simulink library "groundCheckSubsystem"  (R2021b)
settings: Solver=VariableStepAuto  StartTime=0.0  StopTime=10.0  RelTol=1e-3
undefined symbols (not defined in the file): Simulation
settings Model: Creator=mat  LastModifiedBy=mat

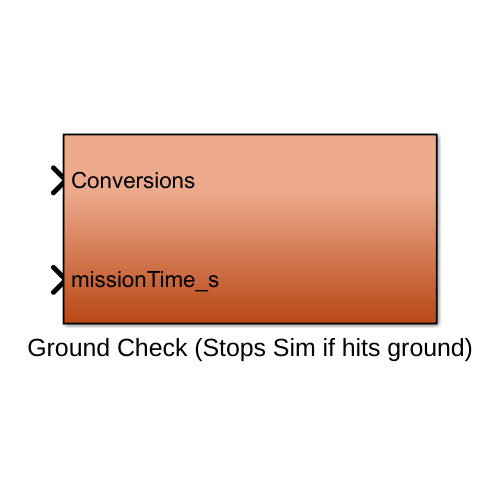
[thumbnail: Simulink's stored preview of the top-level diagram]
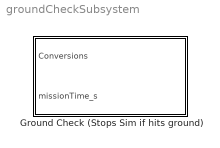
== system groundCheckSubsystem ==
  Ground Check (Stops Sim if hits ground) : Subsystem

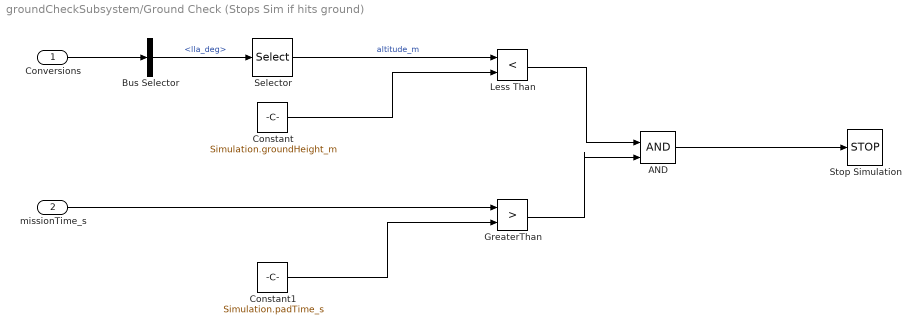
== system groundCheckSubsystem/Ground Check (Stops Sim if hits ground) ==
  Conversions : Inport  OutDataTypeStr=Bus: Conversions_BusType
  missionTime_s : Inport  Port=2
  AND : Logic  IconShape=distinctive  AllPortsSameDT=off  OutDataTypeStr=boolean
  Bus Selector : BusSelector  OutputSignals=lla_deg
  Constant : Constant  Value=Simulation.groundHeight_m
      settings: AttributesFormatString=%<Value>
  Constant1 : Constant  Value=Simulation.padTime_s
      settings: AttributesFormatString=%<Value>
  GreaterThan : RelationalOperator  Operator=>  OutDataTypeStr=boolean  RndMeth=Simplest
  Less Than : RelationalOperator  Operator=<  OutDataTypeStr=boolean  RndMeth=Simplest
  Selector : Selector  InputPortWidth=3  IndexOptions=Index vector (dialog)  Indices=[3]  OutputSizes=1
  Stop Simulation : Stop
  wires:
  AND/1 -> Stop Simulation/1
  GreaterThan/1 -> AND/2
  Less Than/1 -> AND/1
  Constant1/1 -> GreaterThan/2
  missionTime_s/1 -> GreaterThan/1
  Constant/1 -> Less Than/2
  Selector/1 -> Less Than/1  "altitude_m"
  Bus Selector/1 -> Selector/1  "<lla_deg>"
  Conversions/1 -> Bus Selector/1
